simulink model "ap1"  (Simulink 7.1)
settings: Solver=ode45  StartTime=0.0  StopTime=10.0  RelTol=1e-3
settings Model: Creator=madalin  LastModifiedBy=madalin

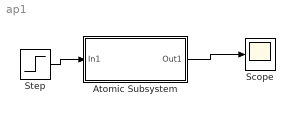
== system ap1 ==
  Atomic Subsystem : Subsystem  TreatAsAtomicUnit=on  mask{a=25}
      mask prompts: a "variabila"
  Scope : Scope
  Step : Step  Time=0  SampleTime=0
  wires:
  Step/1 -> Atomic Subsystem/1(In1)
  Atomic Subsystem/1(Out1) -> Scope/1

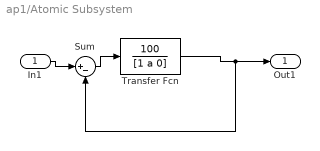
== system ap1/Atomic Subsystem ==
  In1 : Inport  OutDataType=sfix(16)  OutScaling=2^0
  Sum : Sum  Inputs=|+-  OutDataType=sfix(16)  OutScaling=2^0
  Transfer Fcn : TransferFcn  Numerator=100  Denominator=[1 a 0]
  Out1 : Outport  OutDataType=sfix(16)  OutScaling=2^0
  wires:
  Transfer Fcn/1 -> Out1/1, Sum/2
  In1/1 -> Sum/1
  Sum/1 -> Transfer Fcn/1
